simulink model "test_messages_local"  (R2017a)
settings: Solver=FixedStepAuto  StartTime=0.0  StopTime=10.0  FixedStep=0.01  RelTol=1e-3
libraries: simulink x1
settings Model: Creator=aditya  LastModifiedBy=aditya

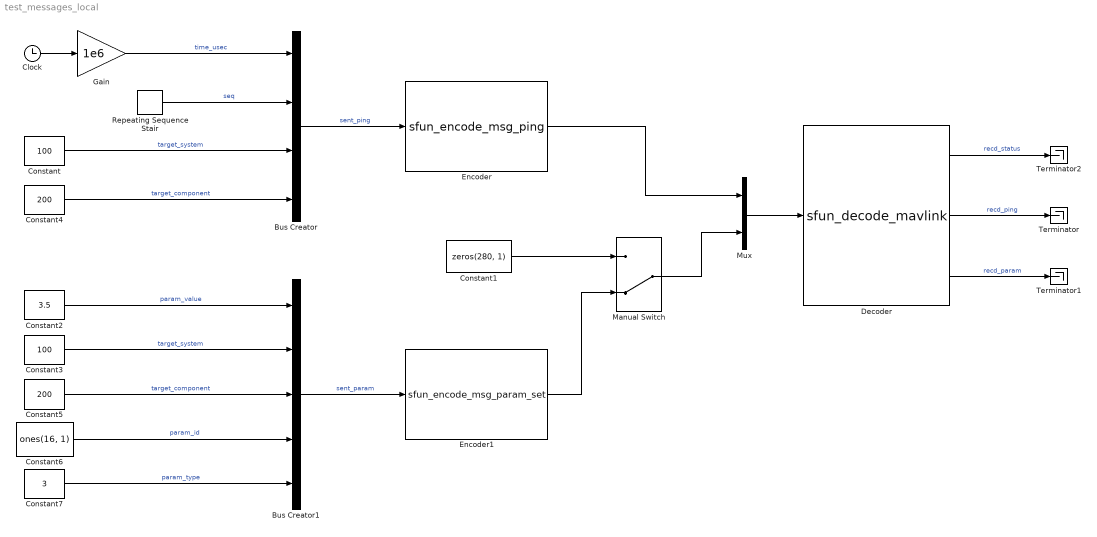
== system test_messages_local ==
  Bus Creator : BusCreator  Inputs=4  OutDataTypeStr=Bus: mavlink_ping_t  NonVirtualBus=on
  Bus Creator1 : BusCreator  Inputs=5  OutDataTypeStr=Bus: mavlink_param_set_t  NonVirtualBus=on
  Clock : Clock
  Constant : Constant  Value=100  OutDataTypeStr=uint8
  Constant1 : Constant  Value=zeros(280, 1)  OutDataTypeStr=uint8
  Constant2 : Constant  Value=3.5  OutDataTypeStr=single
  Constant3 : Constant  Value=100  OutDataTypeStr=uint8
  Constant4 : Constant  Value=200  OutDataTypeStr=uint8
  Constant5 : Constant  Value=200  OutDataTypeStr=uint8
  Constant6 : Constant  Value=ones(16, 1)  OutDataTypeStr=uint8
  Constant7 : Constant  Value=3  OutDataTypeStr=uint8
  Decoder : S-Function  FunctionName=sfun_decode_mavlink  SFunctionDeploymentMode=off  EnableBusSupport=off
  Encoder : S-Function  FunctionName=sfun_encode_msg_ping  SFunctionDeploymentMode=off  EnableBusSupport=off
  Encoder1 : S-Function  FunctionName=sfun_encode_msg_param_set  SFunctionDeploymentMode=off  EnableBusSupport=off
  Gain : Gain  Gain=1e6  OutDataTypeStr=double
  Manual Switch : ManualSwitch  CurrentSetting=0
  Mux : Mux  Inputs=2
  Repeating Sequence Stair : simulink/Sources/Repeating Sequence Stair  OutValues=0:255  tsamp=0.01  OutMin=[]  OutMax=[]  OutDataTypeStr=uint32  OutputDataTypeScalingMode=uint32  OutDataType=fixdt(0,8)  ConRadixGroup=Best Precision: Vector-wise  OutScaling=2^-12
  Terminator : Terminator
  Terminator1 : Terminator
  Terminator2 : Terminator
  wires:
  Bus Creator/1 -> Encoder/1  "sent_ping"
  Clock/1 -> Gain/1
  Gain/1 -> Bus Creator/1  "time_usec"
  Decoder/2 -> Terminator/1  "recd_ping"
  Decoder/3 -> Terminator1/1  "recd_param"
  Encoder/1 -> Mux/1
  Mux/1 -> Decoder/1
  Decoder/1 -> Terminator2/1  "recd_status"
  Repeating Sequence Stair/1 -> Bus Creator/2  "seq"
  Constant/1 -> Bus Creator/3  "target_system"
  Constant4/1 -> Bus Creator/4  "target_component"
  Bus Creator1/1 -> Encoder1/1  "sent_param"
  Constant2/1 -> Bus Creator1/1  "param_value"
  Constant5/1 -> Bus Creator1/3  "target_component"
  Constant3/1 -> Bus Creator1/2  "target_system"
  Constant7/1 -> Bus Creator1/5  "param_type"
  Constant6/1 -> Bus Creator1/4  "param_id"
  Manual Switch/1 -> Mux/2
  Constant1/1 -> Manual Switch/1
  Encoder1/1 -> Manual Switch/2
